simulink library "hduc_lib"  (Simulink 8.7)
settings: Solver=ode45  StartTime=0.0  StopTime=10.0  RelTol=1e-3
undefined symbols (not defined in the file): display, value
libraries: DSPBAPrim x3, DSPBAFilters x2, DSPBABase x2
settings Model: Creator=bigcat  LastModifiedBy=5g

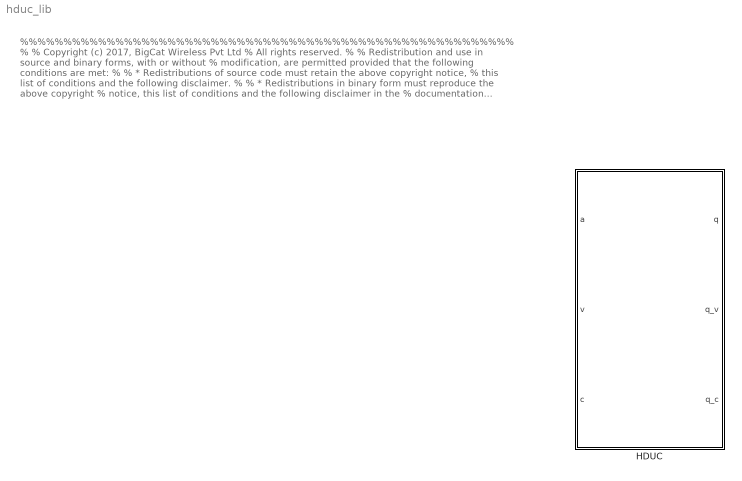
== system hduc_lib ==
  note: %%%%%%%%%%%%%%%%%%%%%%%%%%%%%%%%%%%%%%%%%%%%%%%%%%%%%%%%%
      |  %
      |  % Copyright (c) 2017, BigCat Wireless Pvt Ltd
      |  % All rights reserved.
      |  %
      |  % Redistribution and use in source and binary forms, with or without
      |  % modification, are permitted provided that the following conditions are met:
      |  %
      |  %     * Redistributions of source code must retain the above copyright notice,
      |  %       this list of conditions and the following disclaimer.
      |  %
      |  %     * Redistributions in binary form must reproduce the above copyright
      |  %       notice, this list of conditions and the following disclaimer in the
      |  %       documentation and/or other materials provided with the distribution.
      |  %
      |  %     * Neither the name of the copyright holder nor the names of its contributors
      |  %       may be used to endorse or promote products derived from this software
      |  %       without specific prior written permission.
      |  %
      |  %
      |  %
      |  % THIS SOFTWARE IS PROVIDED BY THE COPYRIGHT HOLDERS AND CONTRIBUTORS "AS IS"
      |  % AND ANY EXPRESS OR IMPLIED WARRANTIES, INCLUDING, BUT NOT LIMITED TO, THE
      |  % IMPLIED WARRANTIES OF MERCHANTABILITY AND FITNESS FOR A PARTICULAR PURPOSE ARE
      |  % DISCLAIMED. IN NO EVENT SHALL THE COPYRIGHT HOLDER OR CONTRIBUTORS BE LIABLE
      |  % FOR ANY DIRECT, INDIRECT, INCIDENTAL, SPECIAL, EXEMPLARY, OR CONSEQUENTIAL
      |  % DAMAGES (INCLUDING, BUT NOT LIMITED TO, PROCUREMENT OF SUBSTITUTE GOODS OR
      |  % SERVICES; LOSS OF USE, DATA, OR PROFITS; OR BUSINESS INTERRUPTION) HOWEVER
      |  % CAUSED AND ON ANY THEORY OF LIABILITY, WHETHER IN CONTRACT, STRICT LIABILITY,
      |  % OR TORT (INCLUDING NEGLIGENCE OR OTHERWISE) ARISING IN ANY WAY OUT OF THE USE
      |  % OF THIS SOFTWARE, EVEN IF ADVISED OF THE POSSIBILITY OF SUCH DAMAGE.
      |  %
      |   %%%%%%%%%%%%%%%%%%%%%%%%%%%%%%%%%%%%%%%%%%%%%%%%%%%%%%
  HDUC : Subsystem  mask{HB_filt_SampleRate=0, HB_filt_Interpolation=0, HB_filt_ChanCount=0, HB_filt_coeffs=fi([zeros(1,15) 0.99 zeros(1,15)],1,16,15), HB_filt_base_addr=0, output_word_length=0, output_fraction_length=0, Multiplication_factor=0, Bits_to_shift_left=0, Pipeline_stages=0, ClockMargin=0}
      mask Display:
      | disp('HDUC');
      | port_label('input',1,'d');
      | port_label('input',2,'v');
      | port_label('input',3,'c');
      | port_label('output',1,'q');
      | port_label('output',2,'q_v');
      | port_label('output',3,'q_c');

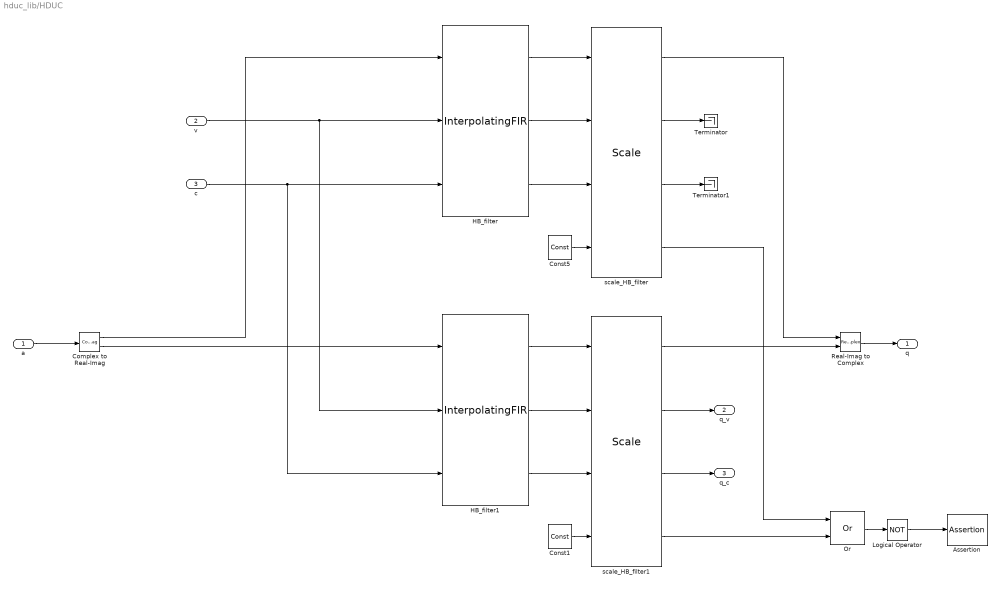
== system hduc_lib/HDUC ==
  a : Inport
  v : Inport  Port=2
  c : Inport  Port=3
  Assertion : Assertion  Enabled=off  AssertionFailFcn=display('Simulation stopped, because an over/underflow was detected in HDDC/HB7')  StopWhenAssertionFail=off
  Complex to Real-Imag : ComplexToRealImag
  Const1 : DSPBAPrim/Const  primtype=const  nInputs=0  nOutputs=1  omode=Inherit via internal rule  otype=sfix(16)  scale=2^-15  rndmethod=Unbiased  factor=1  satmethod=Symmetric  shift_vec=[0 1 2 -1]  value=0  inPortNames=['+'; '+';]  outPortNames=[' ']  dspbaimage=dspba_prim.jpg  text=fprintf('%s', num2str(value));  style=Optimised  visibilities=8 + 1024  floatPrecision=float32_m23  version=20120820
  Const5 : DSPBAPrim/Const  primtype=const  nInputs=0  nOutputs=1  omode=Inherit via internal rule  otype=sfix(16)  scale=2^-15  rndmethod=Unbiased  factor=1  satmethod=Symmetric  shift_vec=[0 1 2 -1]  value=0  inPortNames=['+'; '+';]  outPortNames=[' ']  dspbaimage=dspba_prim.jpg  text=fprintf('%s', num2str(value));  style=Optimised  visibilities=8 + 1024  floatPrecision=float32_m23  version=20120820
  HB_filter : DSPBAFilters/InterpolatingFIR  nInputRate=HB_filt_SampleRate  interp=HB_filt_Interpolation  nchan=HB_filt_ChanCount  symmetry=Symmetrical  coef=HB_filt_coeffs  addr=HB_filt_base_addr  rwmode=Constant  nband=Half Band  exposebus=off  latency=8  version=20090407  recon=off  MM=[0,1,2,3,4,5,6,7,8,9,10,11,12,13,14,15]
  HB_filter1 : DSPBAFilters/InterpolatingFIR  nInputRate=HB_filt_SampleRate  interp=HB_filt_Interpolation  nchan=HB_filt_ChanCount  symmetry=Symmetrical  coef=HB_filt_coeffs  addr=HB_filt_base_addr  rwmode=Constant  nband=Half Band  exposebus=off  latency=8  version=20090407  recon=off  MM=[0,1,2,3,4,5,6,7,8,9,10,11,12,13,14,15]
  Logical Operator : Logic  Operator=NOT  Inputs=1  AllPortsSameDT=off  OutDataTypeStr=boolean
  Or : DSPBAPrim/Or  primtype=or  nInputs=2  nOutputs=1  omode=Inherit via internal rule  otype=sfix(16)  scale=2^-15  rndmethod=Unbiased  factor=1  satmethod=Symmetric  shift_vec=[0 1 2 -1]  value=0  inPortNames=[' '; ' '; ' '; ' '; ' '; ' '; ' '; ' '; ' '; ' '; ' '; ' '; ' '; ' '; ' '; ' '; ]  outPortNames=[' ']  dspbaimage=dspba_prim.jpg  text=fprintf('|');  style=Optimised  visibilities=8+2  version=20090407
  Real-Imag to Complex : RealImagToComplex
  Terminator : Terminator
  Terminator1 : Terminator
  scale_HB_filter : DSPBABase/Scale  otype=sfix(output_word_length)  scale=2^-output_fraction_length  rndmethod=Truncate  factor=Multiplication_factor  satmethod=Symmetric  shift_vec=Bits_to_shift_left  latency=7  wideSimulation=off  version=20090407
  scale_HB_filter1 : DSPBABase/Scale  otype=sfix(output_word_length)  scale=2^-output_fraction_length  rndmethod=Truncate  factor=Multiplication_factor  satmethod=Symmetric  shift_vec=Bits_to_shift_left  latency=7  wideSimulation=off  version=20090407
  q : Outport
  q_v : Outport  Port=2
  q_c : Outport  Port=3
  wires:
  HB_filter/3 -> scale_HB_filter/3
  HB_filter/2 -> scale_HB_filter/2
  HB_filter/1 -> scale_HB_filter/1
  Const5/1 -> scale_HB_filter/4
  scale_HB_filter/4 -> Or/1
  HB_filter1/3 -> scale_HB_filter1/3
  HB_filter1/2 -> scale_HB_filter1/2
  HB_filter1/1 -> scale_HB_filter1/1
  Const1/1 -> scale_HB_filter1/4
  Complex to Real-Imag/2 -> HB_filter1/1
  v/1 -> HB_filter1/2, HB_filter/2
  c/1 -> HB_filter1/3, HB_filter/3
  scale_HB_filter1/1 -> Real-Imag to Complex/2
  scale_HB_filter1/2 -> q_v/1
  scale_HB_filter1/3 -> q_c/1
  scale_HB_filter1/4 -> Or/2
  a/1 -> Complex to Real-Imag/1
  Complex to Real-Imag/1 -> HB_filter/1
  scale_HB_filter/2 -> Terminator/1
  scale_HB_filter/3 -> Terminator1/1
  Real-Imag to Complex/1 -> q/1
  scale_HB_filter/1 -> Real-Imag to Complex/1
  Or/1 -> Logical Operator/1
  Logical Operator/1 -> Assertion/1
